simulink model "Problem1"  (R2020b)
settings: Solver=VariableStepAuto  StartTime=0.0  StopTime=10.0  RelTol=1e-3
settings Model: Creator=Dell  LastModifiedBy=Dell

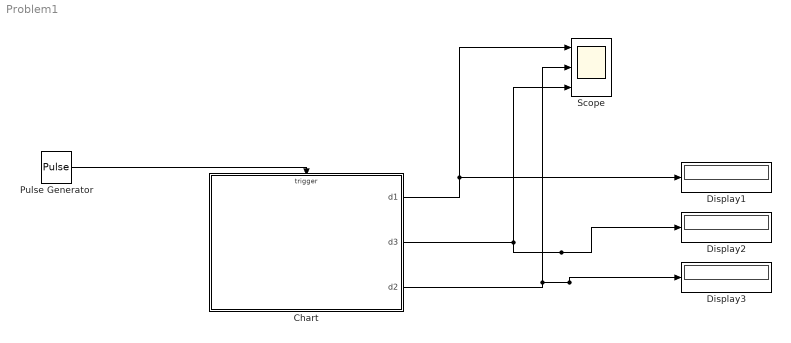
== system Problem1 ==
  Chart : Stateflow chart  TreatAsAtomicUnit=on
  Display1 : Display
  Display2 : Display
  Display3 : Display
  Pulse Generator : DiscretePulseGenerator  PulseType=Time based  Period=1  PulseWidth=50
  Scope : Scope  NumInputPorts=3
  wires:
  Pulse Generator/1 -> Chart/Trigger
  Chart/1(d1) -> Display1/1, Scope/1
  Chart/2(d3) -> Scope/3, Display2/1
  Chart/3(d2) -> Display3/1, Scope/2

== stateflow chart Problem1/Chart ==
  settings: executeAtInitialization=1
  state digit1 [parallel]
    settings: executionOrder=1
    state zero
      en:d1=0;
    state one
      en:d1=1;
    state two
      en:d1=2;
    state three
      en:d1=3;
    state four
      en:d1=4;
    digit1.three -> digit1.four : inputclick
    digit1.one -> digit1.two : inputclick
    digit1.two -> digit1.three : inputclick
    digit1.zero -> digit1.one : inputclick
    (default) -> digit1.zero
    digit1.four -> digit1.zero : inputclick/{digit2.inc2}
  state digit2 [parallel]
    settings: executionOrder=2
    state three
      en:d2=3;
    state two1
      en:d2=2;
    state one
      en:d2=1;
    state zero
      en:d2=0;
    state four
      en:d2=4;
    digit2.three -> digit2.four : inc2
    two1 -> digit2.three : inc2
    digit2.one -> two1 : inc2
    digit2.zero -> digit2.one : inc2
    (default) -> digit2.zero
    digit2.four -> digit2.zero : inc2/{digit3.inc3}
  state digit3 [parallel]
    settings: executionOrder=3
    state three
      en:d3=3;
    state zero1
      en:d3=0;
    state one1
      en:d3=1;
    state two
      en:d3=2;
    state four
      en:d3=4;
    digit3.three -> digit3.four : inc3
    zero1 -> one1 : inc3
    (default) -> zero1
    digit3.two -> digit3.three : inc3
    one1 -> digit3.two : inc3
    digit3.four -> zero1 : inc3
  data: d1 output; d3 output; d2 output
  events: inc2 local FUNCTION_CALL_EVENT; inc3 local FUNCTION_CALL_EVENT; inputclick input RISING_EDGE_EVENT
